simulink model "finalserial_2019b"  (R2019b)
settings: Solver=VariableStepAuto  StartTime=0.0  StopTime=10.0  RelTol=1e-3
libraries: commutil2 x3, xpcutilitieslib x2, commcrc2 x2
settings Model: Creator=JClae  LastModifiedBy=toons

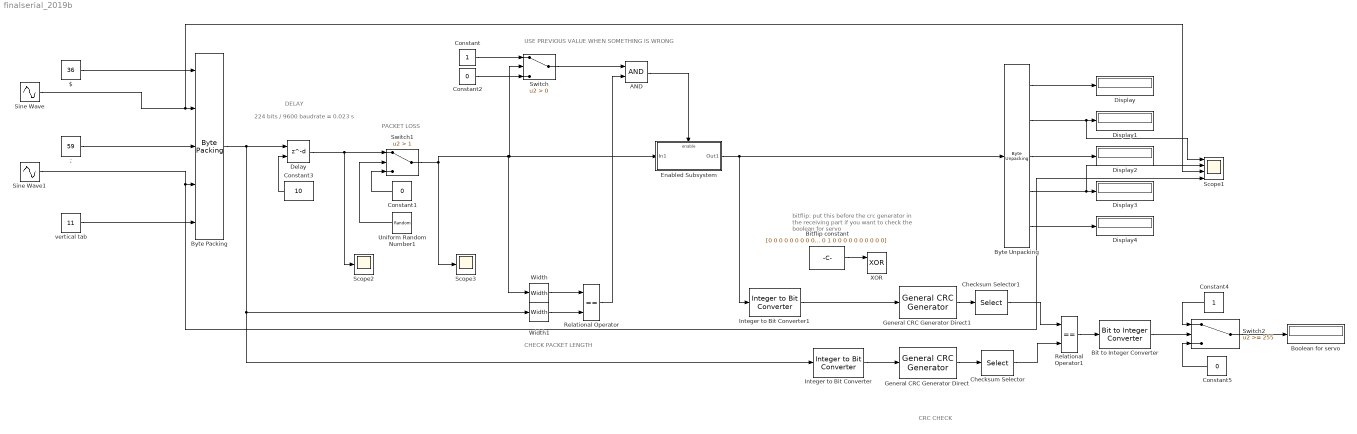
== system finalserial_2019b ==
  note: bitflip: put this before the crc generator
      | in the receiving part if you want to check
      | the boolean for servo
  note: CRC CHECK
  note: 224 bits / 9600 baudrate = 0.023 s
  note: USE PREVIOUS VALUE WHEN SOMETHING IS WRONG
  note: CHECK PACKET LENGTH
  note: PACKET LOSS
  note: DELAY
  $ : Constant  Value=36  OutMin=0  OutMax=360  OutDataTypeStr=single
  ; : Constant  Value=59  OutMin=0  OutMax=255  OutDataTypeStr=single
  AND : Logic  AllPortsSameDT=off  OutDataTypeStr=boolean
  Bit to Integer Converter : commutil2/Bit to Integer Converter  nbits=8  bitOrder=MSB first  signedOutputValues=Unsigned  outDtype=Inherit via internal rule  outDtypeSigned=Inherit via internal rule
  Bitflip constant : Constant  Value=[0 0 0 0 0 0 0 0 0 0 0 0 0 0 0 0 0 0 0 0 0 0 0 0 0 0 0 0 0 0 0 0 0 0 0 0 0 0 0 0 0 0 0 0 0 0 0 0 0 0 0 0 0 0 0 0 0 0 0 0 0 0 0 0 0 0 0 0 0 0 0 0 0 0 0 0 0 0 0 0 0 0 0 0 0 0 0 0 0 0 0 0 0 0 0 0 0 0 0 0 0 0 0 0 0 0 0 0 0 0 0 0 0 0 0 0 0 0 0 0 0 0 0 0 0 0 0 0 0 0 0 0 0 0 0 0 0 0 0 0 0 0 0 0 0 0 0 0 0 0 0 0 0 0 0 0 0 0 0 0 0 0 0 0 0 0 0 0 0 0 0 0 0 0 0 0 0 0 0 0 0 0 0 0 0 0 0 0 0 0 0 0 0 0 0 0 0 0 0 0 0 0 0 0 0 0 0 0 0 0 0 0 0 1 0 0 0 0 0 0 0 0 0 0]
  Boolean for servo : Display
  "Byte Packing " : xpcutilitieslib/Byte Packing   MaskPackedDataType=uint32  MaskUnpackedDataTypes={'single','double','single','double','single'}  MaskAlignment=1
  "Byte Unpacking " : xpcutilitieslib/Byte Unpacking   MaskUnpackedDataTypes={'single','double','single','double','single'}  MaskUnpackedDataSizes={[1],[1],[1],[1],[1]}  MaskAlignment=1
      settings: SourceProductBaseCode=XP
  Checksum Selector : Selector  InputPortWidth=232  IndexOptions=Index vector (dialog)  Indices=(225:232)  OutputSizes=1
  Checksum Selector1 : Selector  InputPortWidth=232  IndexOptions=Index vector (dialog)  Indices=(225:232)  OutputSizes=1
  Constant : Constant
  Constant1 : Constant  Value=0  OutDataTypeStr=int32
  Constant2 : Constant  Value=0
  Constant3 : Constant  Value=10
  Constant4 : Constant
  Constant5 : Constant  Value=0
  Delay : Delay  DelayLengthSource=Input port
      settings: InputPortMap=u0,p1
  Display{,1..4} (5 alike) : Display
  Enabled Subsystem : Subsystem  TreatAsAtomicUnit=on
  General CRC Generator Direct : commcrc2/General CRC Generator  genPoly='z^8 + z^2 + z + 1'  iniStates=1  directMethod=on  reflectInputBytes=off  reflectChecksums=off  finalXOR=1  numChecksums=1
      settings: SourceProductBaseCode=CM
  General CRC Generator Direct1 : commcrc2/General CRC Generator  genPoly='z^8 + z^2 + z + 1'  iniStates=1  directMethod=on  reflectInputBytes=off  reflectChecksums=off  finalXOR=1  numChecksums=1
      settings: SourceProductBaseCode=CM
  Integer to Bit Converter : commutil2/Integer to Bit Converter  nbits=32  signedInputValues=Unsigned  bitOrder=MSB first  outDtype=boolean
  Integer to Bit Converter1 : commutil2/Integer to Bit Converter  nbits=32  signedInputValues=Unsigned  bitOrder=MSB first  outDtype=boolean
  Relational Operator : RelationalOperator  Operator===  OutDataTypeStr=boolean  RndMeth=Simplest
  Relational Operator1 : RelationalOperator  Operator===  OutDataTypeStr=boolean  RndMeth=Simplest
  Scope1 : Scope  NumInputPorts=4
  Scope2 : Scope
  Scope3 : Scope
  Sine Wave : Sin  Amplitude=90  Bias=90  SampleTime=0.05
  Sine Wave1 : Sin  Amplitude=90  Bias=90  Phase=1.57079  SampleTime=0.05
  Switch : Switch  Criteria=u2 > Threshold
  Switch1 : Switch  Criteria=u2 > Threshold  Threshold=1
  Switch2 : Switch  Threshold=255
  Uniform Random Number1 : UniformRandomNumber  Minimum=0  Maximum=100  Seed=5  SampleTime=1/9600
  Width : Width
  Width1 : Width
  XOR : Logic  Operator=XOR  AllPortsSameDT=off  OutDataTypeStr=boolean
  vertical tab : Constant  Value=11  OutMin=0  OutMax=255  OutDataTypeStr=single
  wires:
  $/1 -> "Byte Packing "/1
  ;/1 -> "Byte Packing "/3
  "Byte Unpacking "/3 -> Display2/1
  "Byte Unpacking "/2 -> Scope1/1, Display1/1
  vertical tab/1 -> "Byte Packing "/5
  "Byte Unpacking "/4 -> Scope1/2, Display3/1
  "Byte Unpacking "/5 -> Display4/1
  "Byte Packing "/1 -> Integer to Bit Converter/1, Width1/1, Delay/1
  "Byte Unpacking "/1 -> Display/1
  Switch1/1 -> Width/1, Switch/2, Enabled Subsystem/1(In1), Scope3/1
  Constant1/1 -> Switch1/3
  Uniform Random Number1/1 -> Switch1/2
  Width/1 -> Relational Operator/1
  Width1/1 -> Relational Operator/2
  Enabled Subsystem/1(Out1) -> Integer to Bit Converter1/1, "Byte Unpacking "/1
  Constant/1 -> Switch/1
  Constant2/1 -> Switch/3
  Relational Operator/1 -> AND/2
  Switch/1 -> AND/1
  AND/1 -> Enabled Subsystem/Enable
  Constant3/1 -> Delay/2
  Integer to Bit Converter/1 -> General CRC Generator Direct/1
  General CRC Generator Direct1/1 -> Checksum Selector1/1
  Checksum Selector1/1 -> Relational Operator1/1
  General CRC Generator Direct/1 -> Checksum Selector/1
  Checksum Selector/1 -> Relational Operator1/2
  Bitflip constant/1 -> XOR/1
  Relational Operator1/1 -> Bit to Integer Converter/1
  Bit to Integer Converter/1 -> Switch2/2
  Constant4/1 -> Switch2/1
  Constant5/1 -> Switch2/3
  Switch2/1 -> Boolean for servo/1
  Integer to Bit Converter1/1 -> General CRC Generator Direct1/1
  Sine Wave/1 -> Scope1/3, "Byte Packing "/2
  Sine Wave1/1 -> Scope1/4, "Byte Packing "/4
  Delay/1 -> Switch1/1, Scope2/1

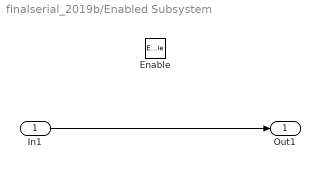
== system finalserial_2019b/Enabled Subsystem ==
  In1 : Inport
  Enable : EnablePort
  Out1 : Outport
  wires:
  In1/1 -> Out1/1
